simulink model "SCARAHybCtrl"  (R2023b)
settings: Solver=VariableStepAuto  StartTime=0.0  StopTime=10.0  RelTol=1e-3
values from neighbouring files (symbols this model uses):
  b1 = L1 / 2    (= 0.2)    [init.m]
  b2 = L2 / 2    (= 0.125)    [init.m]
  dq0 = [0.0; 0.0; 0.0]    [init.m]
  env_damping = 150.0    (= 150)    [init.m]
  env_stiffness = 15000.0    (= 15000)    [init.m]
  friction_coulomb = [0.2; 0.2; 0.05]    [init.m]
  friction_viscous = [0.5; 0.5; 0.1]    [init.m]
  g = 9.807    [init.m]
  I1 = 0.417    [init.m]
  I2 = 0.206    [init.m]
  L1 = 0.4    [init.m]
  L2 = 0.25    [init.m]
  m1 = 29.58    [init.m]
  m2 = 15.0    (= 15)    [init.m]
  m3 = 5.0    (= 5)    [init.m]
  m_load = 6.0    (= 6)    [init.m]
  q0 = [pi/4; pi/4; 0.10]    [init.m]
  z_surface = 0.0    (= 0)    [init.m]
settings Model: Creator=davi_  LastModifiedBy=davi_

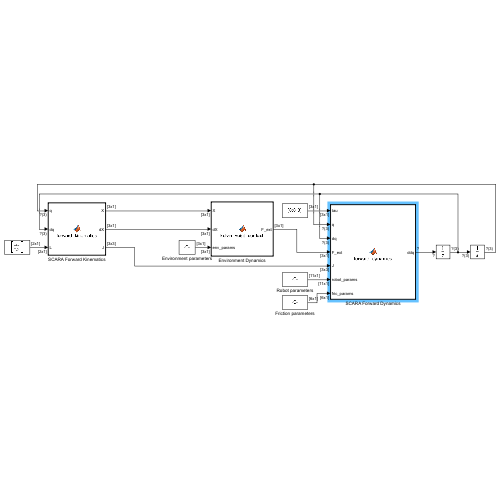
[thumbnail: Simulink's stored preview of the top-level diagram]
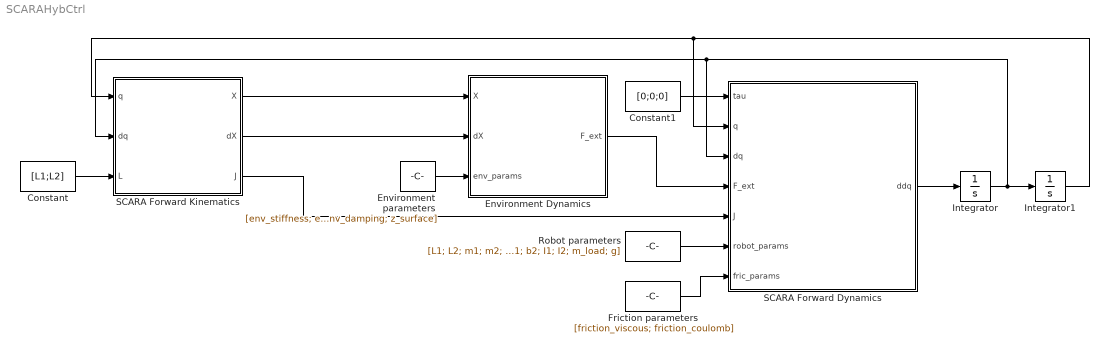
== system SCARAHybCtrl ==
  Constant : Constant  Value=[L1;L2]  VectorParams1D=off
  Constant1 : Constant  Value=[0;0;0]  VectorParams1D=off
  Environment Dynamics : MATLAB Function  TreatAsAtomicUnit=on
  Environment parameters : Constant  Value=[env_stiffness; env_damping; z_surface]  VectorParams1D=off
  Friction parameters : Constant  Value=[friction_viscous; friction_coulomb]  VectorParams1D=off
  Integrator : Integrator  InitialCondition=dq0
  Integrator1 : Integrator  InitialCondition=q0
  Robot parameters : Constant  Value=[L1; L2; m1; m2; m3; b1; b2; I1; I2; m_load; g]  VectorParams1D=off
  SCARA Forward Dynamics : MATLAB Function  TreatAsAtomicUnit=on
  SCARA Forward Kinematics : MATLAB Function  TreatAsAtomicUnit=on
  wires:
  Constant/1 -> SCARA Forward Kinematics/3(L)
  SCARA Forward Kinematics/2(dX) -> Environment Dynamics/2(dX)
  SCARA Forward Kinematics/1(X) -> Environment Dynamics/1(X)
  Environment parameters/1 -> Environment Dynamics/3(env_params)
  Robot parameters/1 -> SCARA Forward Dynamics/6(robot_params)
  Friction parameters/1 -> SCARA Forward Dynamics/7(fric_params)
  SCARA Forward Dynamics/1(ddq) -> Integrator/1
  Integrator/1 -> SCARA Forward Dynamics/3(dq), SCARA Forward Kinematics/2(dq), Integrator1/1
  Integrator1/1 -> SCARA Forward Kinematics/1(q), SCARA Forward Dynamics/2(q)
  SCARA Forward Kinematics/3(J) -> SCARA Forward Dynamics/5(J)
  Environment Dynamics/1(F_ext) -> SCARA Forward Dynamics/4(F_ext)
  Constant1/1 -> SCARA Forward Dynamics/1(tau)

== matlab function SCARAHybCtrl/Environment Dynamics ==
  data: X input; F_ext output; dX input; env_params input
function F_ext = kelvin_voigt_contact(X, dX, env_params)
    % """
    % Computes the external contact force using a unilateral Kelvin-Voigt model.
    %
    % This function simulates a rigid ground surface. It evaluates the current
    % Cartesian position and velocity of the end-effector. If penetration into
    % the surface occurs, it applies a viscoelastic restoring force. The contact
    % is strictly unilateral (the ground can push, but cannot pull).
    %
    % Args:
    %     X (3x1 column vector): Cartesian position of the end-effector [x; y; z].
    %     dX (3x1 column vector): Cartesian velocity of the end-effector [dx; dy; dz].
    %     env_params (3x1 column vector): Environment parameters 
    %                                     [stiffness; damping; z_surface].
    %
    % Returns:
    %     F_ext (3x1 column vector): External force vector applied to the 
    %                                end-effector [Fx; Fy; Fz].
    % """

    % Extract Z-axis states
    z = X(3);
    dz = dX(3);
    
    % Extract environment parameters
    Ke = env_params(1);
    Be = env_params(2);
    z_sup = env_params(3);
    
    % Initialize Z-axis force
    Fz = 0.0;
    
    % Check for penetration (contact condition)
    if z <= z_sup
        % Viscoelastic force: Stiffness * penetration_depth - Damping * velocity
        Fz = Ke * (z_sup - z) - Be * dz;
        
        % Unilateral constraint: The ground cannot pull the end-effector
        if Fz < 0.0
            Fz = 0.0;
        end
    end
    
    % Assemble the 3x1 external force vector (acting only on the Z-axis)
    F_ext = [0.0; 0.0; Fz];

end

== matlab function SCARAHybCtrl/SCARA Forward Kinematics ==
  data: q input; X output; dq input; L input; dX output; J output
function [X, dX, J] = forward_kinematics(q, dq, L)
    % """
    % Computes the forward kinematics and analytical Jacobian for a 3-DOF SCARA.
    %
    % This function calculates the end-effector's Cartesian position, Cartesian 
    % velocity, and the 3x3 analytical Jacobian matrix based on the current 
    % joint configuration. The geometric model is based on a planar 2R 
    % manipulator augmented with a prismatic Z-axis.
    %
    % Args:
    %     q (3x1 column vector): Current joint positions [q1 (rad); q2 (rad); d3 (m)].
    %     dq (3x1 column vector): Current joint velocities [dq1; dq2; dd3].
    %     L (2x1 column vector): Link lengths [L1; L2] in meters.
    %
    % Returns:
    %     X (3x1 column vector): Cartesian position of the end-effector [x; y; z].
    %     dX (3x1 column vector): Cartesian velocity of the end-effector [dx; dy; dz].
    %     J (3x3 matrix): Analytical Jacobian matrix relating joint velocities
    %                     to Cartesian velocities (dX = J * dq).
    % """

    % Extract individual joint variables
    q1 = q(1);
    q2 = q(2);
    q3 = q(3);
    
    % Extract link lengths
    L1 = L(1);
    L2 = L(2);
    
    % Precompute trigonometric terms to optimize simulation speed
    c1 = cos(q1);
    s1 = sin(q1);
    c12 = cos(q1 + q2);
    s12 = sin(q1 + q2);
    
    % 1. Forward Kinematics (Position X)
    x = L1 * c1 + L2 * c12;
    y = L1 * s1 + L2 * s12;
    z = q3;
    
    X = [x; y; z];
    
    % 2. Analytical Jacobian Matrix (J)
    % Row 1: Partial derivatives of x with respect to q1, q2, q3
    J11 = -L1 * s1 - L2 * s12;
    J12 = -L2 * s12;
    J13 = 0.0;
    
    % Row 2: Partial derivatives of y with respect to q1, q2, q3
    J21 = L1 * c1 + L2 * c12;
    J22 = L2 * c12;
    J23 = 0.0;
    
    % Row 3: Partial derivatives of z with respect to q1, q2, q3
    J31 = 0.0;
    J32 = 0.0;
    J33 = 1.0;
    
    J = [J11, J12, J13;
         J21, J22, J23;
         J31, J32, J33];
         
    % 3. Cartesian Velocity (dX)
    dX = J * dq;

end

== matlab function SCARAHybCtrl/SCARA Forward Dynamics ==
  data: tau input; ddq output; q input; dq input; F_ext input; J input; robot_params input; fric_params input
function ddq = forward_dynamics(tau, q, dq, F_ext, J, robot_params, fric_params)
    % """
    % Computes the forward dynamics of the 3-DOF SCARA robot.
    %
    % This function calculates the joint accelerations (ddq) given the applied
    % joint torques, current states, external contact forces, and the analytical
    % Jacobian. The dynamic model uses equations exactly derived from Massaro
    % et al. (2023) for the planar 2R components, augmented with a decoupled
    % Z-axis prismatic dynamic model.
    %
    % Args:
    %     tau (3x1 column vector): Control torques applied to joints [Nm; Nm; N].
    %     q (3x1 column vector): Current joint positions [q1; q2; d3].
    %     dq (3x1 column vector): Current joint velocities [dq1; dq2; dd3].
    %     F_ext (3x1 column vector): External forces from the environment [Fx; Fy; Fz].
    %     J (3x3 matrix): Analytical Jacobian matrix.
    %     robot_params (11x1 column vector): Physical parameters array.
    %     fric_params (6x1 column vector): Friction parameters array.
    %
    % Returns:
    %     ddq (3x1 column vector): Joint accelerations [ddq1; ddq2; ddd3].
    % """

    % 1. Extract Parameters
    L1 = robot_params(1); L2 = robot_params(2);
    m1 = robot_params(3); m2 = robot_params(4); m3 = robot_params(5);
    b1 = robot_params(6); b2 = robot_params(7);
    I1 = robot_params(8); I2 = robot_params(9);
    M_load = robot_params(10);
    g = robot_params(11);
    
    B_visc = fric_params(1:3);
    F_coulomb = fric_params(4:6);

    % 2. Extract States and Precompute Trigonometry
    q1 = q(1); 
    q2 = q(2);
    dq1 = dq(1); 
    dq2 = dq(2); 
    
    c2 = cos(q2);
    s2 = sin(q2);

    % 3. Inertia Matrix M(q) (Massaro et al. 2023, Eqs. 14-16, h1=h2=0)
    m11 = I1 + I2 + m1*(b1^2) + m2*(L1^2 + b2^2 + 2*L1*b2*c2) + ...
          M_load*(L1^2 + L2^2 + 2*L1*L2*c2);
          
    m12 = I2 + m2*(b2^2 + L1*b2*c2) + M_load*(L2^2 + L1*L2*c2);
    
    m22 = I2 + m2*(b2^2) + M_load*(L2^2);
    
    % Z-axis inertia (decoupled RRP)
    m33 = m3 + M_load;
    
    M_matrix = [m11, m12, 0.0;
                m12, m22, 0.0;
                0.0, 0.0, m33];

    % 4. Coriolis and Centrifugal Vector C(q, dq)*dq (Massaro Eq. 13)
    % Note: Using s2 (sin(q2)) for Coriolis terms as per standard 2R dynamics
    c1 = -L1 * dq2 * (2*dq1 + dq2) * (m2*b2*s2 + M_load*L2*s2);
    c2 = L1 * (dq1^2) * (m2*b2*s2 + M_load*L2*s2);
    
    C_vector = [c1; c2; 0.0];

    % 5. Gravity Vector G(q)
    % Assuming Z-axis points upwards, gravity acts downwards
    G_vector = [0.0; 0.0; m33 * g];

    % 6. Friction Torque Vector
    % Models viscous and Coulomb friction. A small deadzone can be used in 
    % sign() to avoid numerical chattering at exactly zero velocity if needed.
    tau_fric = B_visc .* dq + F_coulomb .* sign(dq);

    % 7. Solve Forward Dynamics for Joint Accelerations (ddq)
    % Equation: M*ddq + C + G + tau_fric = tau - J' * F_ext
    % Therefore: ddq = M \ (tau - C - G - tau_fric - J' * F_ext)
    
    rhs = tau - C_vector - G_vector - tau_fric - (J' * F_ext);
    
    % Using mldivide (\) for efficient matrix inversion
    ddq = M_matrix \ rhs;

end
